simulink model "Scheduler"  (R2015a)
settings: Solver=ode45  StartTime=0.0  StopTime=10.0  RelTol=1e-3
libraries: simulink x1
settings Model: Creator=Morya  LastModifiedBy=Morya

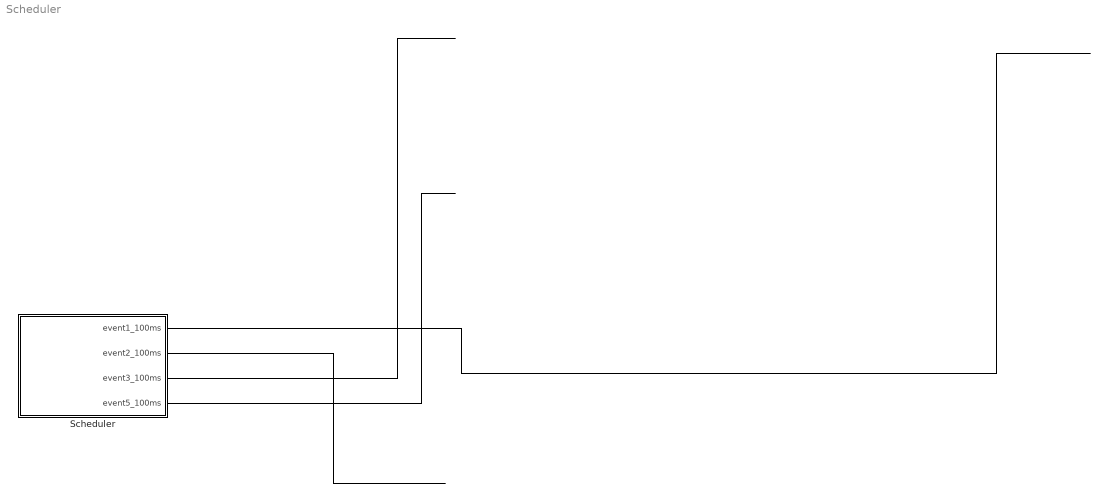
== system Scheduler ==
  "Scheduler " : Subsystem
  wires:
  "Scheduler "/1(event1_100ms) -> ?
  "Scheduler "/2(event2_100ms) -> ?
  "Scheduler "/3("event3_100ms ") -> ?
  "Scheduler "/4("event5_100ms ") -> ?

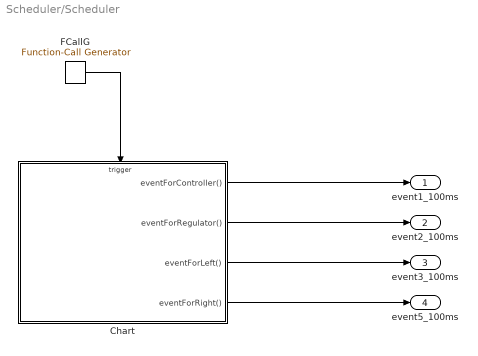
== system Scheduler/Scheduler  ==
  Chart : Stateflow chart  TreatAsAtomicUnit=on
  FCallG : simulink/Ports & Subsystems/Function-Call Generator  sample_time=0.1  numberOfIterations=1
  event1_100ms : Outport
  event2_100ms : Outport  Port=2
  "event3_100ms " : Outport  Port=3
  "event5_100ms " : Outport  Port=4
  wires:
  Chart/1(eventForController()) -> event1_100ms/1
  Chart/2(eventForRegulator()) -> event2_100ms/1
  Chart/3(eventForLeft()) -> "event3_100ms "/1
  FCallG/1 -> Chart/Trigger
  Chart/4(eventForRight()) -> "event5_100ms "/1

== stateflow chart Scheduler/Scheduler /Chart ==
  state Start
    on every(1,fCallG): send(eventForController);
    on every(1,fCallG): send(eventForRegulator);
    on every(1,fCallG): send(eventForLeft);
    on every(1,fCallG): send(eventForRight);
  (default) -> Start
  events: fCallG input FUNCTION_CALL_EVENT; eventForController output FUNCTION_CALL_EVENT; eventForRegulator output FUNCTION_CALL_EVENT; eventForLeft output FUNCTION_CALL_EVENT; eventForRight output FUNCTION_CALL_EVENT
